simulink model "prsig_2"  (Simulink 5.0)
settings: Solver=ode45  StartTime=0.0  StopTime=10.0  RelTol=1e-3
undefined symbols (not defined in the file): get
libraries: dsparch4 x1, simulink x1, dspsnks4 x1
settings Model: LastModifiedBy=zilic

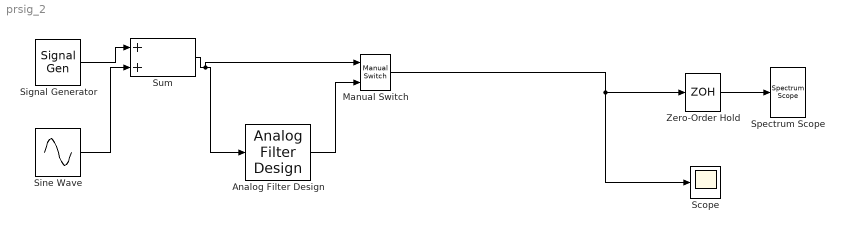
== system prsig_2 ==
  Analog Filter Design : dsparch4/Analog Filter Design  method=Chebyshev II  filttype=Lowpass  N=8  Wlo=2*pi*30  Whi=2*pi*20  Rp=2  Rs=40
  Manual Switch : simulink/Signal Routing/Manual Switch  sw=1  action=0
  Scope : Scope
  Signal Generator : SignalGenerator  WaveForm=square  Amplitude=4  Frequency=5
  Sine Wave : Sin  Frequency=2*pi*22  SampleTime=0
  Spectrum Scope : dspsnks4/Spectrum Scope  ScopeProperties=off  Domain=Frequency  HorizSpan=1  UseBuffer=on  BufferSize=256  Overlap=128  inpFftLenInherit=off  FFTlength=128  numAvg=2  DisplayProperties=off  AxisGrid=on  Memory=off  FrameNumber=on  AxisLegend=off  AxisZoom=off  OpenScopeAtSimStart=on  OpenScopeImmediately=off  FigPos=get(0,'defaultfigureposition')  AxisProperties=on  XUnits=Hertz  XRange=[0...Fs/2]  InheritXIncr=on  XIncr=1.0  XLabel=Samples  YUnits=dB  YLabel=Magnitude, dB  LineProperties=off
      settings: YMin=0.8756298067581  YMax=35.1300303186128
  Sum : Sum  Inputs=|++  SaturateOnIntegerOverflow=on
  Zero-Order Hold : ZeroOrderHold  SampleTime=1/200
  wires:
  Signal Generator/1 -> Sum/1
  Sine Wave/1 -> Sum/2
  Analog Filter Design/1 -> Manual Switch/2
  Zero-Order Hold/1 -> Spectrum Scope/1
  Sum/1 -> Analog Filter Design/1, Manual Switch/1
  Manual Switch/1 -> Zero-Order Hold/1, Scope/1
